simulink model "example"  (R2019b)
settings: Solver=VariableStepAuto  StartTime=0.0  StopTime=10.0  RelTol=1e-3
undefined symbols (not defined in the file or in its folder): ContractBlock, ContractGuaranteeBlock, ContractValidatorBlock
libraries: simulink x2, CoCoSTLib x1
settings Model: Creator=xiayu  LastModifiedBy=xiayu

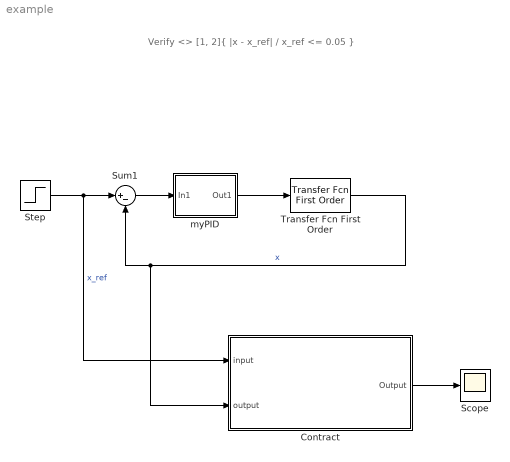
== system example ==
  note: Verify
      | <> [1, 2]{ |x - x_ref| / x_ref <= 0.05 }
  Contract : Subsystem  mask(ContractBlock){ContractBlockType=ContractBlock, ShowInLibBrowser=on}
      mask init:
      | set_param(gcb, 'LinkStatus', 'none');
      settings: CopyFcn=set_param(gcb, 'LinkStatus', 'none');
      mask DialogControl DescTextVar Prompt: Contract block
      mask Display: text(0.5, 0.5, '{\bf\fontsize{20}Contract}', 'hor', 'center', 'texmode','on');
  Scope : Scope
  Step : Step  After=10  SampleTime=0
  Sum1 : Sum  Inputs=|+-
  Transfer Fcn First Order : simulink/Discrete/Transfer Fcn First Order  PoleZ=0.95  ICPrevOutput=0.0  DoSatur=off
      settings: SourceProductName=Simulink
  myPID : Subsystem
  wires:
  myPID/1(Out1) -> Transfer Fcn First Order/1
  Transfer Fcn First Order/1 -> Contract/2(output), Sum1/2  "x"
  Sum1/1 -> myPID/1(In1)
  Step/1 -> Contract/1(input), Sum1/1  "x_ref"
  Contract/1(Output) -> Scope/1

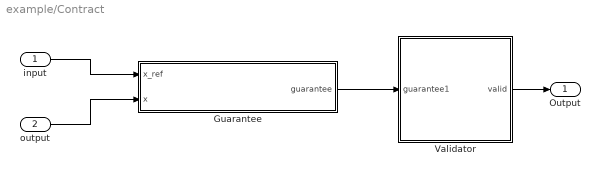
== system example/Contract ==
  input : Inport
  output : Inport  Port=2
  Guarantee : Subsystem  mask(ContractGuaranteeBlock){ContractBlockType=ContractGuaranteeBlock}
      mask init:
      | set_param(gcb, 'LinkStatus', 'none');
      mask DialogControl DescTextVar Prompt: Guarantee block
      mask Display: text(0.5, 0.5, '{\bf\fontsize{20}Guarantee}', 'hor', 'center', 'texmode','on');
  Validator : Subsystem  mask(ContractValidatorBlock){assumePorts=0, guaranteePorts=1, modePorts=0, ContractBlockType=ContractValidatorBlock}
      mask prompts: assumePorts "Assume ports     :"; guaranteePorts "Guarantee ports :"; modePorts "Mode ports        :"
      mask help: The validator block implements the following logic: <br> <br> <b>Sofar</b>(assume<sub>1</sub> <b>&#8743;</b> assume<sub>2</sub> <b>&#8743;</b> ... assume<sub>k</sub>) <b>&rarr;</b> <b>Sofar</b>(guarantee<sub>1</sub> <b>&#8743;</b> guarantee<sub>2</sub> <b>&#8743;</b> ... guarantee<sub>m</sub> <b>&#8743;</b> mode<sub>1</sub> <b>&#8743;</b> mode<sub>2</sub> <b>&#8743;</b> ... <b>&#8743;</b> mode<sub>n</sub> )<br> where mode<sub>i</sub> = require<sub>i</sub> <b>&rarr;</b> ensure<sub>i</sub>
      mask init:
      | set_param(gcb,'LinkStatus','none');
      | try
      | coco_blockCallbacks.CoCoSimContract.validatorCallback(gcb);
      | catch
      | end
      mask Display: disp(' ')
  Output : Outport
  wires:
  Guarantee/1(guarantee) -> Validator/1(guarantee1)
  input/1 -> Guarantee/1(x_ref)
  output/1 -> Guarantee/2(x)
  Validator/1(valid) -> Output/1

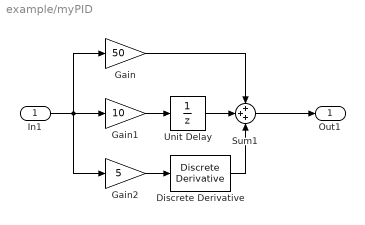
== system example/myPID ==
  In1 : Inport
  Discrete Derivative : simulink/Discrete/Discrete Derivative  gainval=1.0  ICPrevScaledInput=0.0  OutMin=[]  OutMax=[]  OutDataType=fixdt(1, 16)  OutScaling=2^-10  DoSatur=off
  Gain : Gain  Gain=50
  Gain1 : Gain  Gain=10
  Gain2 : Gain  Gain=5
  Sum1 : Sum  Inputs=+++
  Unit Delay : UnitDelay  SampleTime=-1  HasFrameUpgradeWarning=on
  Out1 : Outport
  wires:
  Discrete Derivative/1 -> Sum1/3
  Unit Delay/1 -> Sum1/2
  Gain/1 -> Sum1/1
  In1/1 -> Gain2/1, Gain/1, Gain1/1
  Sum1/1 -> Out1/1
  Gain1/1 -> Unit Delay/1
  Gain2/1 -> Discrete Derivative/1

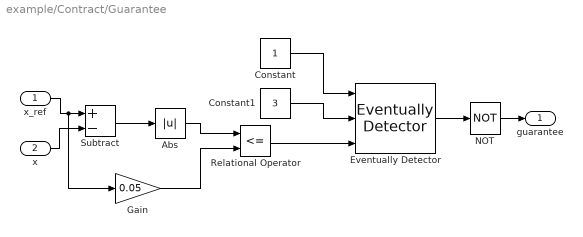
== system example/Contract/Guarantee ==
  x_ref : Inport
  x : Inport  Port=2
  Abs : Abs
  Constant : Constant
  Constant1 : Constant  Value=3
  "Eventually Detector " : CoCoSTLib/Operators-Detectors/Eventually Detector   SystemSampleTime=-1  Latency=0  AutoFrameSizeCalculation=off
      settings: SourceProductName=CoCoSTLib
  Gain : Gain  Gain=0.05
  NOT : Logic  Operator=NOT  IconShape=distinctive  AllPortsSameDT=off  OutDataTypeStr=boolean
  Relational Operator : RelationalOperator  Operator=<=  OutDataTypeStr=boolean  RndMeth=Simplest
  Subtract : Sum  Inputs=+-
  guarantee : Outport  OutDataTypeStr=boolean  VectorParamsAs1DForOutWhenUnconnected=off
  wires:
  x_ref/1 -> Gain/1, Subtract/1
  x/1 -> Subtract/2
  Subtract/1 -> Abs/1
  Abs/1 -> Relational Operator/1
  Gain/1 -> Relational Operator/2
  Relational Operator/1 -> "Eventually Detector "/3
  Constant/1 -> "Eventually Detector "/1
  Constant1/1 -> "Eventually Detector "/2
  "Eventually Detector "/1 -> NOT/1
  NOT/1 -> guarantee/1

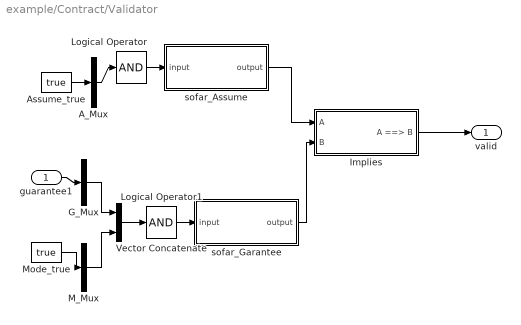
== system example/Contract/Validator ==
  guarantee1 : Inport  OutDataTypeStr=boolean  PortDimensions=1
  A_Mux : Mux  Inputs=1
  Assume_true : Constant  Value=true  OutDataTypeStr=boolean
  G_Mux : Mux  Inputs=1
  Implies : Subsystem
  Logical Operator : Logic  Inputs=1  AllPortsSameDT=off  OutDataTypeStr=boolean
  Logical Operator1 : Logic  Inputs=1  AllPortsSameDT=off  OutDataTypeStr=boolean
  M_Mux : Mux  Inputs=1
  Mode_true : Constant  Value=true  OutDataTypeStr=boolean
  Vector Concatenate : Concatenate
  sofar_Assume : Subsystem
  sofar_Garantee : Subsystem
  valid : Outport  VectorParamsAs1DForOutWhenUnconnected=off
  wires:
  sofar_Assume/1(output) -> Implies/1(A)
  sofar_Garantee/1(output) -> Implies/2(B)
  Implies/1(A ==> B) -> valid/1
  A_Mux/1 -> Logical Operator/1
  Logical Operator/1 -> sofar_Assume/1(input)
  Logical Operator1/1 -> sofar_Garantee/1(input)
  G_Mux/1 -> Vector Concatenate/1
  guarantee1/1 -> G_Mux/1
  Vector Concatenate/1 -> Logical Operator1/1
  M_Mux/1 -> Vector Concatenate/2
  Assume_true/1 -> A_Mux/1
  Mode_true/1 -> M_Mux/1

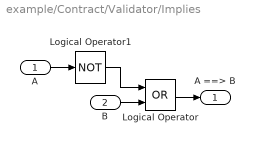
== system example/Contract/Validator/Implies ==
  A : Inport
  B : Inport  Port=2
  Logical Operator : Logic  Operator=OR  AllPortsSameDT=off  OutDataTypeStr=boolean
  Logical Operator1 : Logic  Operator=NOT  AllPortsSameDT=off  OutDataTypeStr=boolean
  A ==> B : Outport  VectorParamsAs1DForOutWhenUnconnected=off
  wires:
  Logical Operator1/1 -> Logical Operator/1
  A/1 -> Logical Operator1/1
  Logical Operator/1 -> A ==> B/1
  B/1 -> Logical Operator/2

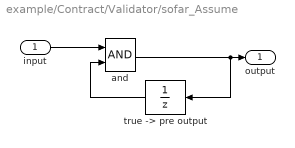
== system example/Contract/Validator/sofar_Assume ==
  input : Inport  OutDataTypeStr=boolean
  and : Logic  AllPortsSameDT=off  OutDataTypeStr=boolean
  "true -> pre output" : UnitDelay  InitialCondition=true  SampleTime=-1  HasFrameUpgradeWarning=on
  output : Outport  OutDataTypeStr=boolean  VectorParamsAs1DForOutWhenUnconnected=off
  wires:
  input/1 -> and/1
  "true -> pre output"/1 -> and/2
  and/1 -> "true -> pre output"/1, output/1

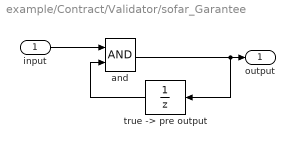
== system example/Contract/Validator/sofar_Garantee ==
  input : Inport  OutDataTypeStr=boolean
  and : Logic  AllPortsSameDT=off  OutDataTypeStr=boolean
  "true -> pre output" : UnitDelay  InitialCondition=true  SampleTime=-1  HasFrameUpgradeWarning=on
  output : Outport  OutDataTypeStr=boolean  VectorParamsAs1DForOutWhenUnconnected=off
  wires:
  input/1 -> and/1
  "true -> pre output"/1 -> and/2
  and/1 -> "true -> pre output"/1, output/1
